simulink model "Factorial"  (R2017b)
settings: Solver=FixedStepDiscrete  StartTime=0.0  StopTime=10.0  RelTol=1e-3
settings Model: Creator=Hady Sallam  LastModifiedBy=Hady Sallam
settings OptimizationCC: DefaultParameterBehavior=Inlined  PassReuseOutputArgsAs=Individual arguments
settings DebuggingCC: ParameterTunabilityLossMsg=error
settings SFSimCC: MATLABDynamicMemAlloc=off
settings RTWCC: SystemTargetFile=ert.tlc  GenCodeOnly=on  TemplateMakefile=ert_default_tmf  GenerateReport=on  IncludeHyperlinkInReport=on  LaunchReport=on  GenerateTraceInfo=on  GenerateTraceReport=on  GenerateTraceReportSl=on  GenerateTraceReportSf=on  GenerateTraceReportEml=on
settings CodeAppCC: ForceParamTrailComments=on  IgnoreCustomStorageClasses=off  OperatorAnnotations=on  SimulinkDataObjDesc=on  SFDataObjDesc=on  InsertBlockDesc=on
settings ERTTargetCC: TargetLangStandard=C99 (ISO)  GenerateSampleERTMain=on  InlinedParameterPlacement=NonHierarchical  ERTCustomFileTemplate=example_file_process.tlc  EnableUserReplacementTypes=on

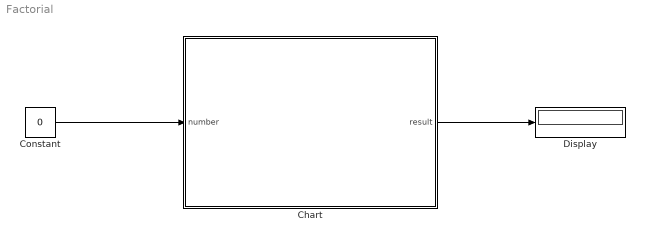
== system Factorial ==
  Chart : Stateflow chart  TreatAsAtomicUnit=on
  Constant : Constant  Value=0
  Display : Display
  wires:
  Constant/1 -> Chart/1(number)
  Chart/1(result) -> Display/1

== stateflow chart Factorial/Chart ==
  (default) -> (junction 21)
  (junction 21) -> (junction 23) [order 2] : [number == 0]
  (junction 23) -> (junction 26)
  (junction 21) -> (junction 1) [order 1] : [number > 0]
  (junction 1) -> (junction 3) : {index = number;
      | result = 1;}
  (junction 3) -> (junction 5) [order 1] : [index > 0 & number != 0]
  (junction 5) -> (junction 7) : {result = result * index;}
  (junction 7) -> (junction 3) : {index = index - 1}
  (junction 3) -> (junction 10) [order 2]
  (junction 26) -> (junction 10)
  data: number input double; index local double; result output double
